simulink model "controller_v12_pagani_zonda_R"  (R2022b)
settings: Solver=ode4  StartTime=0.0  StopTime=10  FixedStep=0.00001  RelTol=1e-3
values from neighbouring files (symbols this model uses):
  m = 6    [coordinator_v2.m]
  N = 10    [coordinator_v2.m]
undefined symbols (not defined in the file or in its folder): PD_result, sd, X, Y, Z
libraries: sm_lib x235, nesl_utility x83
(part 5 of 5)

== system controller_v12_pagani_zonda_R/Subsystem/base ==
  ReferenceFrame : sm_lib/Frames and Transforms/Reference Frame
  Visual : sm_lib/Body Elements/Brick Solid  GraphicAmbientColor=[0.15 0.15 0.15 1.0]  BasedOnType=Density  BrickDimensions=[0.001, 0.001, 0.001]  BrickDimensionUnits=m  CenterOfMass=[0, 0, 0]  CenterOfMassUnits=m  GraphicDiffuseColor=[0.5, 0.5, 0.5]  Density=1000  DensityUnits=kg/m^3  DoExposeReferenceFrame=on  GraphicEmissiveColor=[0.0 0.0 0.0 1.0]  ExportEntireGeometry=off  SerializedFrames=<Frames/>  MarkerShape=Sphere  MarkerSize=10  GraphicType=FromGeometry  InertiaType=Custom  Mass=0  MassUnits=kg  MomentsOfInertia=[0, 0, 0]  MomentsOfInertiaUnits=kg*m^2  GraphicOpacity=1  ProductsOfInertia=[0, 0, 0]  ProductsOfInertiaUnits=kg*m^2  GraphicShininess=75  GraphicSpecularColor=[0.5 0.5 0.5 1.0]  GraphicVisPropType=SimpleVisualProperties
  VisualOriginTransform : sm_lib/Frames and Transforms/Rigid Transform  TranslationMethod=Cartesian  TranslationStandardOffset=0  TranslationLengthUnit=m  TranslationStandardAxis=+Z  TranslationCartesianOffset=[0, 0, 0]  TranslationROffset=0  TranslationROffsetUnits=m  TranslationZOffset=0  TranslationZOffsetUnits=m  TranslationThetaOffset=0  TranslationThetaOffsetUnits=deg  RotationMethod=RotationSequence  RotationAngleUnits=deg  RotationStandardAxis=+Z  RotationAngle=0.0  RotationArbitraryAxis=[0 0 1]  FollAlignAxisA=+X  BaseAlignAxisA=+Y  FollAlignAxisB=+Y  BaseAlignAxisB=+Z  RotationSequenceAxes=BaseAxes  RotationSequence=XYZ  RotationSequenceAngles=[0, 0, 0]  RotationSequenceAnglesUnits=rad  RotationMatrix=[1 0 0; 0 1 0; 0 0 1]  Quaternion=[1 0 0 0]
  floating_base_OriginTransform : sm_lib/Frames and Transforms/Rigid Transform  TranslationMethod=Cartesian  TranslationStandardOffset=0  TranslationLengthUnit=m  TranslationStandardAxis=+Z  TranslationCartesianOffset=[0, 0, 0]  TranslationROffset=0  TranslationROffsetUnits=m  TranslationZOffset=0  TranslationZOffsetUnits=m  TranslationThetaOffset=0  TranslationThetaOffsetUnits=deg  RotationMethod=RotationSequence  RotationAngleUnits=deg  RotationStandardAxis=+Z  RotationAngle=0.0  RotationArbitraryAxis=[0 0 1]  FollAlignAxisA=+X  BaseAlignAxisA=+Y  FollAlignAxisB=+Y  BaseAlignAxisB=+Z  RotationSequenceAxes=BaseAxes  RotationSequence=XYZ  RotationSequenceAngles=[0, 0, 0]  RotationSequenceAnglesUnits=rad  RotationMatrix=[1 0 0; 0 1 0; 0 0 1]  Quaternion=[1 0 0 0]
  F : PMIOPort  Side=Left
  F1 : PMIOPort  Port=2  Side=Right
  connections:
  VisualOriginTransform/LConn1 -- ReferenceFrame/RConn1 -- F/RConn1 -- floating_base_OriginTransform/LConn1
  Visual/RConn1 -- VisualOriginTransform/RConn1
  floating_base_OriginTransform/RConn1 -- F1/RConn1

== system controller_v12_pagani_zonda_R/Subsystem/imu_link ==
  Inertia : sm_lib/Body Elements/Inertia  InertiaType=Custom  Mass=0.001  MassUnits=kg  CenterOfMass=[0, 0, 0]  CenterOfMassUnits=m  MomentsOfInertia=[0.0001, 0.0001, 0.0001]  MomentsOfInertiaUnits=kg*m^2  ProductsOfInertia=[0, 0, 0]  ProductsOfInertiaUnits=kg*m^2  GraphicType=None  MarkerShape=Inertia  MarkerSize=20  GraphicVisPropType=SimpleVisualProperties  GraphicDiffuseColor=[0.5 0.5 0.5]  GraphicSpecularColor=[0.5 0.5 0.5 1.0]  GraphicAmbientColor=[0.15 0.15 0.15 1.0]  GraphicEmissiveColor=[0.0 0.0 0.0 1.0]  GraphicShininess=75  GraphicOpacity=1.0
  InertiaOriginTransform : sm_lib/Frames and Transforms/Rigid Transform  TranslationMethod=Cartesian  TranslationStandardOffset=0  TranslationLengthUnit=m  TranslationStandardAxis=+Z  TranslationCartesianOffset=[0, 0, 0]  TranslationROffset=0  TranslationROffsetUnits=m  TranslationZOffset=0  TranslationZOffsetUnits=m  TranslationThetaOffset=0  TranslationThetaOffsetUnits=deg  RotationMethod=RotationSequence  RotationAngleUnits=deg  RotationStandardAxis=+Z  RotationAngle=0.0  RotationArbitraryAxis=[0 0 1]  FollAlignAxisA=+X  BaseAlignAxisA=+Y  FollAlignAxisB=+Y  BaseAlignAxisB=+Z  RotationSequenceAxes=BaseAxes  RotationSequence=XYZ  RotationSequenceAngles=[0, 0, 0]  RotationSequenceAnglesUnits=rad  RotationMatrix=[1 0 0; 0 1 0; 0 0 1]  Quaternion=[1 0 0 0]
  ReferenceFrame : sm_lib/Frames and Transforms/Reference Frame
  Visual : sm_lib/Body Elements/Brick Solid  GraphicAmbientColor=[0.15 0.15 0.15 1.0]  BasedOnType=Density  BrickDimensions=[0.001, 0.001, 0.001]  BrickDimensionUnits=m  CenterOfMass=[0, 0, 0]  CenterOfMassUnits=m  GraphicDiffuseColor=[0.8, 0, 0]  Density=1000  DensityUnits=kg/m^3  DoExposeReferenceFrame=on  GraphicEmissiveColor=[0.0 0.0 0.0 1.0]  ExportEntireGeometry=off  SerializedFrames=<Frames/>  MarkerShape=Sphere  MarkerSize=10  GraphicType=FromGeometry  InertiaType=Custom  Mass=0  MassUnits=kg  MomentsOfInertia=[0, 0, 0]  MomentsOfInertiaUnits=kg*m^2  GraphicOpacity=1  ProductsOfInertia=[0, 0, 0]  ProductsOfInertiaUnits=kg*m^2  GraphicShininess=75  GraphicSpecularColor=[0.5 0.5 0.5 1.0]  GraphicVisPropType=SimpleVisualProperties
  VisualOriginTransform : sm_lib/Frames and Transforms/Rigid Transform  TranslationMethod=Cartesian  TranslationStandardOffset=0  TranslationLengthUnit=m  TranslationStandardAxis=+Z  TranslationCartesianOffset=[0, 0, 0]  TranslationROffset=0  TranslationROffsetUnits=m  TranslationZOffset=0  TranslationZOffsetUnits=m  TranslationThetaOffset=0  TranslationThetaOffsetUnits=deg  RotationMethod=RotationSequence  RotationAngleUnits=deg  RotationStandardAxis=+Z  RotationAngle=0.0  RotationArbitraryAxis=[0 0 1]  FollAlignAxisA=+X  BaseAlignAxisA=+Y  FollAlignAxisB=+Y  BaseAlignAxisB=+Z  RotationSequenceAxes=BaseAxes  RotationSequence=XYZ  RotationSequenceAngles=[0, 0, 0]  RotationSequenceAnglesUnits=rad  RotationMatrix=[1 0 0; 0 1 0; 0 0 1]  Quaternion=[1 0 0 0]
  F : PMIOPort  Side=Left
  connections:
  Inertia/RConn1 -- InertiaOriginTransform/RConn1
  ReferenceFrame/RConn1 -- InertiaOriginTransform/LConn1 -- VisualOriginTransform/LConn1 -- F/RConn1
  Visual/RConn1 -- VisualOriginTransform/RConn1

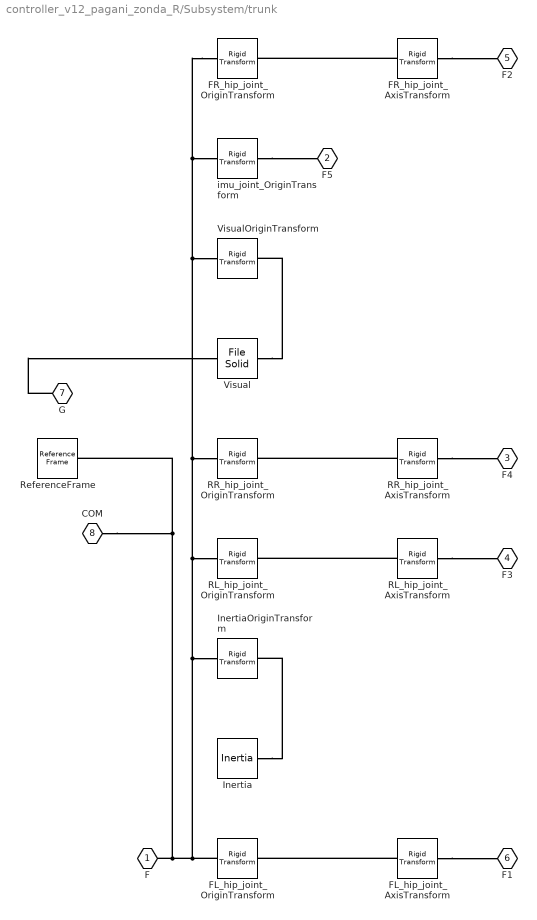
== system controller_v12_pagani_zonda_R/Subsystem/trunk ==
  FL_hip_joint_AxisTransform : sm_lib/Frames and Transforms/Rigid Transform  TranslationMethod=Cartesian  TranslationStandardOffset=0  TranslationLengthUnit=m  TranslationStandardAxis=+Z  TranslationCartesianOffset=[0, 0, 0]  TranslationROffset=0  TranslationROffsetUnits=m  TranslationZOffset=0  TranslationZOffsetUnits=m  TranslationThetaOffset=0  TranslationThetaOffsetUnits=deg  RotationMethod=ArbitraryAxis  RotationAngleUnits=rad  RotationStandardAxis=+Z  RotationAngle=1.570796326794897  RotationArbitraryAxis=[-0, 1, 0]  FollAlignAxisA=+X  BaseAlignAxisA=+Y  FollAlignAxisB=+Y  BaseAlignAxisB=+Z  RotationSequenceAxes=FollowerAxes  RotationSequence=XYX  RotationSequenceAngles=[0 0 0]  RotationSequenceAnglesUnits=deg  RotationMatrix=[1 0 0; 0 1 0; 0 0 1]  Quaternion=[1 0 0 0]
  FL_hip_joint_OriginTransform : sm_lib/Frames and Transforms/Rigid Transform  TranslationMethod=Cartesian  TranslationStandardOffset=0  TranslationLengthUnit=m  TranslationStandardAxis=+Z  TranslationCartesianOffset=[0.1805, 0.047, 0]  TranslationROffset=0  TranslationROffsetUnits=m  TranslationZOffset=0  TranslationZOffsetUnits=m  TranslationThetaOffset=0  TranslationThetaOffsetUnits=deg  RotationMethod=RotationSequence  RotationAngleUnits=deg  RotationStandardAxis=+Z  RotationAngle=0.0  RotationArbitraryAxis=[0 0 1]  FollAlignAxisA=+X  BaseAlignAxisA=+Y  FollAlignAxisB=+Y  BaseAlignAxisB=+Z  RotationSequenceAxes=BaseAxes  RotationSequence=XYZ  RotationSequenceAngles=[0, 0, 0]  RotationSequenceAnglesUnits=rad  RotationMatrix=[1 0 0; 0 1 0; 0 0 1]  Quaternion=[1 0 0 0]
  FR_hip_joint_AxisTransform : sm_lib/Frames and Transforms/Rigid Transform  TranslationMethod=Cartesian  TranslationStandardOffset=0  TranslationLengthUnit=m  TranslationStandardAxis=+Z  TranslationCartesianOffset=[0, 0, 0]  TranslationROffset=0  TranslationROffsetUnits=m  TranslationZOffset=0  TranslationZOffsetUnits=m  TranslationThetaOffset=0  TranslationThetaOffsetUnits=deg  RotationMethod=ArbitraryAxis  RotationAngleUnits=rad  RotationStandardAxis=+Z  RotationAngle=1.570796326794897  RotationArbitraryAxis=[-0, 1, 0]  FollAlignAxisA=+X  BaseAlignAxisA=+Y  FollAlignAxisB=+Y  BaseAlignAxisB=+Z  RotationSequenceAxes=FollowerAxes  RotationSequence=XYX  RotationSequenceAngles=[0 0 0]  RotationSequenceAnglesUnits=deg  RotationMatrix=[1 0 0; 0 1 0; 0 0 1]  Quaternion=[1 0 0 0]
  FR_hip_joint_OriginTransform : sm_lib/Frames and Transforms/Rigid Transform  TranslationMethod=Cartesian  TranslationStandardOffset=0  TranslationLengthUnit=m  TranslationStandardAxis=+Z  TranslationCartesianOffset=[0.1805, -0.047, 0]  TranslationROffset=0  TranslationROffsetUnits=m  TranslationZOffset=0  TranslationZOffsetUnits=m  TranslationThetaOffset=0  TranslationThetaOffsetUnits=deg  RotationMethod=RotationSequence  RotationAngleUnits=deg  RotationStandardAxis=+Z  RotationAngle=0.0  RotationArbitraryAxis=[0 0 1]  FollAlignAxisA=+X  BaseAlignAxisA=+Y  FollAlignAxisB=+Y  BaseAlignAxisB=+Z  RotationSequenceAxes=BaseAxes  RotationSequence=XYZ  RotationSequenceAngles=[0, 0, 0]  RotationSequenceAnglesUnits=rad  RotationMatrix=[1 0 0; 0 1 0; 0 0 1]  Quaternion=[1 0 0 0]
  Inertia : sm_lib/Body Elements/Inertia  InertiaType=Custom  Mass=6  MassUnits=kg  CenterOfMass=[0, 0, 0]  CenterOfMassUnits=m  MomentsOfInertia=[0.0158533, 0.0377999, 0.0456542]  MomentsOfInertiaUnits=kg*m^2  ProductsOfInertia=[-2.75e-05, -6.109999999999999e-05, -3.66e-05]  ProductsOfInertiaUnits=kg*m^2  GraphicType=None  MarkerShape=Inertia  MarkerSize=20  GraphicVisPropType=SimpleVisualProperties  GraphicDiffuseColor=[0.5 0.5 0.5]  GraphicSpecularColor=[0.5 0.5 0.5 1.0]  GraphicAmbientColor=[0.15 0.15 0.15 1.0]  GraphicEmissiveColor=[0.0 0.0 0.0 1.0]  GraphicShininess=75  GraphicOpacity=1.0
  InertiaOriginTransform : sm_lib/Frames and Transforms/Rigid Transform  TranslationMethod=Cartesian  TranslationStandardOffset=0  TranslationLengthUnit=m  TranslationStandardAxis=+Z  TranslationCartesianOffset=[0, 0.0041, -0.0005]  TranslationROffset=0  TranslationROffsetUnits=m  TranslationZOffset=0  TranslationZOffsetUnits=m  TranslationThetaOffset=0  TranslationThetaOffsetUnits=deg  RotationMethod=RotationSequence  RotationAngleUnits=deg  RotationStandardAxis=+Z  RotationAngle=0.0  RotationArbitraryAxis=[0 0 1]  FollAlignAxisA=+X  BaseAlignAxisA=+Y  FollAlignAxisB=+Y  BaseAlignAxisB=+Z  RotationSequenceAxes=BaseAxes  RotationSequence=XYZ  RotationSequenceAngles=[0, 0, 0]  RotationSequenceAnglesUnits=rad  RotationMatrix=[1 0 0; 0 1 0; 0 0 1]  Quaternion=[1 0 0 0]
  RL_hip_joint_AxisTransform : sm_lib/Frames and Transforms/Rigid Transform  TranslationMethod=Cartesian  TranslationStandardOffset=0  TranslationLengthUnit=m  TranslationStandardAxis=+Z  TranslationCartesianOffset=[0, 0, 0]  TranslationROffset=0  TranslationROffsetUnits=m  TranslationZOffset=0  TranslationZOffsetUnits=m  TranslationThetaOffset=0  TranslationThetaOffsetUnits=deg  RotationMethod=ArbitraryAxis  RotationAngleUnits=rad  RotationStandardAxis=+Z  RotationAngle=1.570796326794897  RotationArbitraryAxis=[-0, 1, 0]  FollAlignAxisA=+X  BaseAlignAxisA=+Y  FollAlignAxisB=+Y  BaseAlignAxisB=+Z  RotationSequenceAxes=FollowerAxes  RotationSequence=XYX  RotationSequenceAngles=[0 0 0]  RotationSequenceAnglesUnits=deg  RotationMatrix=[1 0 0; 0 1 0; 0 0 1]  Quaternion=[1 0 0 0]
  RL_hip_joint_OriginTransform : sm_lib/Frames and Transforms/Rigid Transform  TranslationMethod=Cartesian  TranslationStandardOffset=0  TranslationLengthUnit=m  TranslationStandardAxis=+Z  TranslationCartesianOffset=[-0.1805, 0.047, 0]  TranslationROffset=0  TranslationROffsetUnits=m  TranslationZOffset=0  TranslationZOffsetUnits=m  TranslationThetaOffset=0  TranslationThetaOffsetUnits=deg  RotationMethod=RotationSequence  RotationAngleUnits=deg  RotationStandardAxis=+Z  RotationAngle=0.0  RotationArbitraryAxis=[0 0 1]  FollAlignAxisA=+X  BaseAlignAxisA=+Y  FollAlignAxisB=+Y  BaseAlignAxisB=+Z  RotationSequenceAxes=BaseAxes  RotationSequence=XYZ  RotationSequenceAngles=[0, 0, 0]  RotationSequenceAnglesUnits=rad  RotationMatrix=[1 0 0; 0 1 0; 0 0 1]  Quaternion=[1 0 0 0]
  RR_hip_joint_AxisTransform : sm_lib/Frames and Transforms/Rigid Transform  TranslationMethod=Cartesian  TranslationStandardOffset=0  TranslationLengthUnit=m  TranslationStandardAxis=+Z  TranslationCartesianOffset=[0, 0, 0]  TranslationROffset=0  TranslationROffsetUnits=m  TranslationZOffset=0  TranslationZOffsetUnits=m  TranslationThetaOffset=0  TranslationThetaOffsetUnits=deg  RotationMethod=ArbitraryAxis  RotationAngleUnits=rad  RotationStandardAxis=+Z  RotationAngle=1.570796326794897  RotationArbitraryAxis=[-0, 1, 0]  FollAlignAxisA=+X  BaseAlignAxisA=+Y  FollAlignAxisB=+Y  BaseAlignAxisB=+Z  RotationSequenceAxes=FollowerAxes  RotationSequence=XYX  RotationSequenceAngles=[0 0 0]  RotationSequenceAnglesUnits=deg  RotationMatrix=[1 0 0; 0 1 0; 0 0 1]  Quaternion=[1 0 0 0]
  RR_hip_joint_OriginTransform : sm_lib/Frames and Transforms/Rigid Transform  TranslationMethod=Cartesian  TranslationStandardOffset=0  TranslationLengthUnit=m  TranslationStandardAxis=+Z  TranslationCartesianOffset=[-0.1805, -0.047, 0]  TranslationROffset=0  TranslationROffsetUnits=m  TranslationZOffset=0  TranslationZOffsetUnits=m  TranslationThetaOffset=0  TranslationThetaOffsetUnits=deg  RotationMethod=RotationSequence  RotationAngleUnits=deg  RotationStandardAxis=+Z  RotationAngle=0.0  RotationArbitraryAxis=[0 0 1]  FollAlignAxisA=+X  BaseAlignAxisA=+Y  FollAlignAxisB=+Y  BaseAlignAxisB=+Z  RotationSequenceAxes=BaseAxes  RotationSequence=XYZ  RotationSequenceAngles=[0, 0, 0]  RotationSequenceAnglesUnits=rad  RotationMatrix=[1 0 0; 0 1 0; 0 0 1]  Quaternion=[1 0 0 0]
  ReferenceFrame : sm_lib/Frames and Transforms/Reference Frame
  Visual : sm_lib/Body Elements/File Solid  ExtGeomFileName=a1_description\meshes\trunk.stl  UnitType=Custom  ExtGeomFileUnits=m  StepReaderType=HEX  ExportConvexHullGeometry=on  InertiaType=Custom  Mass=0  MassUnits=kg  CenterOfMass=[0, 0, 0]  CenterOfMassUnits=m  MomentsOfInertia=[0, 0, 0]  MomentsOfInertiaUnits=kg*m^2  ProductsOfInertia=[0, 0, 0]  ProductsOfInertiaUnits=kg*m^2  BasedOnType=DensityFromFile  Density=1000  DensityUnits=kg/m^3  DoExposeReferenceFrame=on  SerializedFrames=<Frames/>  GraphicType=FromGeometry  MarkerShape=Sphere  MarkerSize=10  GraphicVisPropType=SimpleVisualProperties  GraphicDiffuseColor=[1, 0.423529411765, 0.0392156862745]  GraphicSpecularColor=[0.5 0.5 0.5 1.0]  GraphicAmbientColor=[0.15 0.15 0.15 1.0]  GraphicEmissiveColor=[0.0 0.0 0.0 1.0]  GraphicShininess=75  GraphicOpacity=1
  VisualOriginTransform : sm_lib/Frames and Transforms/Rigid Transform  TranslationMethod=Cartesian  TranslationStandardOffset=0  TranslationLengthUnit=m  TranslationStandardAxis=+Z  TranslationCartesianOffset=[0, 0, 0]  TranslationROffset=0  TranslationROffsetUnits=m  TranslationZOffset=0  TranslationZOffsetUnits=m  TranslationThetaOffset=0  TranslationThetaOffsetUnits=deg  RotationMethod=RotationSequence  RotationAngleUnits=deg  RotationStandardAxis=+Z  RotationAngle=0.0  RotationArbitraryAxis=[0 0 1]  FollAlignAxisA=+X  BaseAlignAxisA=+Y  FollAlignAxisB=+Y  BaseAlignAxisB=+Z  RotationSequenceAxes=BaseAxes  RotationSequence=XYZ  RotationSequenceAngles=[0, 0, 0]  RotationSequenceAnglesUnits=rad  RotationMatrix=[1 0 0; 0 1 0; 0 0 1]  Quaternion=[1 0 0 0]
  imu_joint_OriginTransform : sm_lib/Frames and Transforms/Rigid Transform  TranslationMethod=Cartesian  TranslationStandardOffset=0  TranslationLengthUnit=m  TranslationStandardAxis=+Z  TranslationCartesianOffset=[0, 0, 0]  TranslationROffset=0  TranslationROffsetUnits=m  TranslationZOffset=0  TranslationZOffsetUnits=m  TranslationThetaOffset=0  TranslationThetaOffsetUnits=deg  RotationMethod=RotationSequence  RotationAngleUnits=deg  RotationStandardAxis=+Z  RotationAngle=0.0  RotationArbitraryAxis=[0 0 1]  FollAlignAxisA=+X  BaseAlignAxisA=+Y  FollAlignAxisB=+Y  BaseAlignAxisB=+Z  RotationSequenceAxes=BaseAxes  RotationSequence=XYZ  RotationSequenceAngles=[0, 0, 0]  RotationSequenceAnglesUnits=rad  RotationMatrix=[1 0 0; 0 1 0; 0 0 1]  Quaternion=[1 0 0 0]
  F : PMIOPort  Side=Left
  F5 : PMIOPort  Port=2  Side=Right
  F4 : PMIOPort  Port=3  Side=Right
  F3 : PMIOPort  Port=4  Side=Right
  F2 : PMIOPort  Port=5  Side=Right
  F1 : PMIOPort  Port=6  Side=Right
  G : PMIOPort  Port=7  Side=Right
  COM : PMIOPort  Port=8  Side=Right
  connections:
  FL_hip_joint_AxisTransform/RConn1 -- F1/RConn1
  FL_hip_joint_AxisTransform/LConn1 -- FL_hip_joint_OriginTransform/RConn1
  FR_hip_joint_AxisTransform/RConn1 -- F2/RConn1
  FR_hip_joint_AxisTransform/LConn1 -- FR_hip_joint_OriginTransform/RConn1
  Inertia/RConn1 -- InertiaOriginTransform/RConn1
  RL_hip_joint_AxisTransform/RConn1 -- F3/RConn1
  RL_hip_joint_AxisTransform/LConn1 -- RL_hip_joint_OriginTransform/RConn1
  RR_hip_joint_AxisTransform/RConn1 -- F4/RConn1
  RR_hip_joint_AxisTransform/LConn1 -- RR_hip_joint_OriginTransform/RConn1
  FR_hip_joint_OriginTransform/LConn1 -- FL_hip_joint_OriginTransform/LConn1 -- COM/RConn1 -- ReferenceFrame/RConn1 -- F/RConn1 -- InertiaOriginTransform/LConn1 -- RL_hip_joint_OriginTransform/LConn1 -- RR_hip_joint_OriginTransform/LConn1 -- VisualOriginTransform/LConn1 -- imu_joint_OriginTransform/LConn1
  Visual/RConn1 -- VisualOriginTransform/RConn1
  imu_joint_OriginTransform/RConn1 -- F5/RConn1
  G/RConn1 -- Visual/LConn1

== matlab function controller_v12_pagani_zonda_R/MATLAB Function ==
  data: q1 input; q2 input; q3 input; q4 input; q5 input; q6 input; q7 input; q8 input; q9 input; q10 input; q11 input; q12 input; w1 input; w2 input; w3 input; w4 input; w5 input; w6 input; w7 input; w8 input; w9 input; w10 input; w11 input; w12 input; ss input; rr input; rl input; fr input; fl input; t input; u1 output; u2 output; u3 output; u4 output; u5 output; u6 output; u7 output; u8 output; u9 output; u10 output; u11 output; u12 output; vrr input; vrl input; vfr input; vfl input; last_MPC_result input; last_PD_result input; update_MPC_result output; MPC_thred input; update_MPC_thred output; update_PD_result output; PD_thred input; update_PD_thred output; sd input; update_sd output
function [u1, u2, u3, u4, u5, u6, u7, u8, u9, u10, u11, u12, update_MPC_result, update_MPC_thred, update_PD_result, update_PD_thred, update_sd] = coordinator(q1, q2, q3, q4, q5, q6, q7, q8, q9, q10, q11, q12, w1, w2, w3, w4, w5, w6, w7, w8, w9, w10, w11, w12, ss, rr, rl, fr, fl, t, vrr, vrl, vfr, vfl, last_MPC_result, last_PD_result, MPC_thred, PD_thred, sd)
    stand_interval = [0; 2];
    q = [q1;q2;q3;q4;q5;q6;q7;q8;q9;q10;q11;q12]; % Joint variable
    cur_time = t - stand_interval(2); % relative time bw world time and standing end time
    N = 10;
    dt = 0.05;
    dt_pd = 0.25;
    v_d = 0.5;
    robot_height = 0.3;
    p_direction = [1; 0; 0]; % direction of movement, must have x^2 + y^2 + z^2 = 1
    update_MPC_thred = MPC_thred;
    update_PD_thred = PD_thred;
    update_sd = sd;

    if cur_time < 0 % running pd controller for standing
        [u1,u2,u3,u4,u5,u6,u7,u8,u9,u10,u11,u12] = PD_constrol_standing(t,q1,q2,q3,q4,q5,q6,q7,q8,q9,q10,q11,q12,w1,w2,w3,w4,w5,w6,w7,w8,w9,w10,w11,w12);
        update_MPC_result = zeros(12, 1);
        update_PD_result = zeros(24, 10);
    else % running mpc controller for nbody motion and PD controller for swing legs after standing period
        if cur_time >= MPC_thred % update foot force every dt after standing end time
            update_MPC_thred = MPC_thred + dt;
            r = [fl; fr; rl; rr]; % Current foot position
%             sd = [0.1902;-0.0072; 0.29; 0; 0; 0; 0; 0; 0; 0; 0; 0; 9.81];
%             sd(7:9) = v_d * p_direction;
%             sd(1:3) = sd(1:3) + (v_d * p_direction) * dt;
%             update_sd = sd;
            sd = updatesd(ss, sd, t, v_d, p_direction, N, dt, robot_height, r);
            update_sd = sd;

            [update_MPC_result, modelist] = MPC_cntr_wrapper(ss, cur_time, r, dt, N, sd);
            y = update_MPC_result;
            [u1mpc,u2mpc,u3mpc,u4mpc,u5mpc,u6mpc,u7mpc,u8mpc,u9mpc,u10mpc,u11mpc,u12mpc] = force2torque(q,y,ss);
        else
            y = last_MPC_result;
            update_MPC_result = last_MPC_result;
            [u1mpc,u2mpc,u3mpc,u4mpc,u5mpc,u6mpc,u7mpc,u8mpc,u9mpc,u10mpc,u11mpc,u12mpc] = force2torque(q,y,ss);
        end

        n = 10; % number of division in swinging period.
        if cur_time >= PD_thred % Call PD function to swing leg every 0.15s
            update_PD_thred = PD_thred + dt_pd;
            r = [fl; fr; rl; rr]; % Current foot position
            vr = [vfl; vfr; vrl; vrr]; % current foot velovity
            [Pfoot_d,Vfoot_d] = get_Traj(cur_time, r, vr, ss, dt_pd, v_d, p_direction, n); % Calculate the desired position of foot at next period according to foot pos and COM pos & velo
            update_PD_result = [Pfoot_d;Vfoot_d]; % Update desired pos & velo for PD control
        else
            Pfoot_d = last_PD_result(1:12,:);
            Vfoot_d = last_PD_result(13:24,:);
            update_PD_result = last_PD_result;
            r = [fl; fr; rl; rr]; % Current foot position
            vr = [vfl; vfr; vrl; vrr]; % current foot velovity
        end

        i = floor(mod(cur_time,dt_pd)/0.025) + 1;

        iteration = floor(mod(cur_time/dt,N));
        if iteration < N/2 % foot 1, 4 on ground

            Pfoot_d(4:6,i) = next_foot_location(2, v_d * p_direction, r, N/2 * dt, n, (N/2), cur_time, N/2 * dt / n, ss);
            Pfoot_d(7:9,i) = next_foot_location(3, v_d * p_direction, r, N/2 * dt, n, N/2, cur_time, N/2 * dt / n, ss);
        else % foot 2, 3 on ground
            Pfoot_d(1:3,i) = next_foot_location(1, v_d * p_direction, r, N/2 * dt, n, N/2, cur_time, N/2 * dt / n, ss);
            Pfoot_d(10:12,i) = next_foot_location(4, v_d * p_direction, r, N/2 * dt, n, N/2, cur_time, N/2 * dt / n, ss);
        end
%         disp(Pfoot_d(:, i), [3, 4]);
%         disp(Vfoot_d(:, i), [3, 4]);
        F_swing = pd_control_for_leg_swing(Vfoot_d(:,i),Pfoot_d(:,i),r,vr); % Calculate the virtual force used for swing legs
        
%         if iteration < N/2 % foot 1, 4 on ground
%             F_swing(1:3) = zeros(3,1); % Forces applied on leg 1 is zero
%             F_swing(10:12) = zeros(3,1);
%         else % foot 2, 3 on ground
%             F_swing(4:6) = zeros(3,1); % Forces applied on leg 1 is zero
%             F_swing(7:9) = zeros(3,1);
%         end




        [u1pd, u2pd, u3pd, u4pd, u5pd, u6pd, u7pd, u8pd, u9pd, u10pd, u11pd, u12pd] = force2torque(q,F_swing,ss);
        
        
        u1 = u1mpc + u1pd;
        u2 = u2mpc + u2pd;
        u3 = u3mpc + u3pd;
        u4 = u4mpc + u4pd;
        u5 = u5mpc + u5pd;
        u6 = u6mpc + u6pd;
        u7 = u7mpc + u7pd;
        u8 = u8mpc + u8pd;
        u9 = u9mpc + u9pd;
        u10 = u10mpc + u10pd;
        u11 = u11mpc + u11pd;
        u12 = u12mpc + u12pd;
    end
end

%% desired system state update
function update = updatesd(ss, sd, t, v_d, p_direction, N, dt, robot_height, r)
        % change p_direction and baseline
        iteration = floor(mod(t/dt,N));
        if iteration < N/2
            front = r(1:3);
            rear = r(9:12);
            fheight = r(3);
            rheight = r(12);
        else
            front = r(4:6);
            rear = r(6:9);
            fheight = r(6);
            rheight = r(9);
        end
        angle = 0;
        if fheight - rheight > 0.1
            slope = (front(3) - rear(3)) / (front(1) - rear(1));
            angle = atan(slope) / 2;
%             sd(1) = (front(1) + rear(1)) / 2 - robot_height * sin(angle);
            sd(1) = (front(1) + rear(1)) / 2;
            sd(3) = robot_height * cos(angle) + (fheight + rheight) / 2;
            sd(5) = -angle;
%             disp(iteration < N/2);
%             disp(transpose(p_direction));
%             disp(transpose(sd));
%             disp(transpose(ss));
        end

        p_direction(1) = cos(angle);
        p_direction(2) = 0;
        p_direction(3) = sin(angle);
        % change sd base on direction
        if t > 1.06 
            sd(5) = -0.1;
        end
        sd(7:9) = [v_d; 0; v_d * tan(angle)];
        sd(1:3) = sd(1:3) + [v_d; 0; v_d * tan(angle)] * dt;
        update = sd;


end
%% PD controller for Standing
function [u1,u2,u3,u4,u5,u6,u7,u8,u9,u10,u11,u12] = PD_constrol_standing(t,q1,q2,q3,q4,q5,q6,q7,q8,q9,q10,q11,q12,w1,w2,w3,w4,w5,w6,w7,w8,w9,w10,w11,w12)
    kp1 = 100;
    kv1 = 40;
    kp2 = 120;
    kv2 = 50;

    q1d = 0; 
    q4d = 0;
    q7d = 0;
    q10d = 0;
    q2d = 0.78;
    q5d = 0.78;
    q8d = 0.78;
    q11d = 0.78;
    q3d = -1.57;
    q6d = -1.57;
    q9d = -1.57;
    q12d = -1.57;

     w1d = 0;
    w2d = 0;
    w3d = 0;
    w4d = 0;
    w5d = 0;
    w6d = 0;
    w7d = 0;
    w8d = 0;
    w9d = 0;
    w10d = 0;
    w11d = 0;
    w12d = 0;

    if t < 0.4
        u1 = 0;
        u2 = 0;
        u3 = 0;
        u4 = 0;
        u5 = 0;
        u6 = 0;
        u7 = 0;
        u8 = 0;
        u9 = 0;
        u10 = 0;
        u11 = 0;
        u12 = 0;
    
    else 
        u1 = kp2*(q1d-q1)+kv2*(w1d-w1);
        u2 = kp2*(q2d-q2)+kv2*(w2d-w2);
        u3 = kp2*(q3d-q3)+kv2*(w3d-w3);
        u4 = kp2*(q4d-q4)+kv2*(w4d-w4);
        u5 = kp2*(q5d-q5)+kv2*(w5d-w5);
        u6 = kp2*(q6d-q6)+kv2*(w6d-w6);
        u7 = kp1*(q7d-q7)+kv1*(w7d-w7);
        u8 = kp1*(q8d-q8)+kv1*(w8d-w8);
        u9 = kp1*(q9d-q9)+kv1*(w9d-w9);
        u10 = kp1*(q10d-q10)+kv1*(w10d-w10);
        u11 = kp1*(q11d-q11)+kv1*(w11d-w11);
        u12 = kp1*(q12d-q12)+kv1*(w12d-w12);
    end
end

%% MPC controller
% Input:
% System state: s, (12, 1)
% time: t
% mode: mode, indicating which foot on ground
% foot positions: r = [r_front_left; r_front_right; r_rear_left;
% r_rear_right]
% Inertial of body: Ib
% body mass: m
% time step: dt
% MPC horizon length: N
% Desired system state: sd
% Output:
% Foot force: y = [F_front_left; F_front_right; F_rear_left;
% F_rear_right]: 
% q: [x; y; z; roll; pitch; yaw; dx; dy; dz; w]
% sd: [xd; yd; zd; roll_d; pitch_d; yaw_d; dx_d; dy_d; dz_d; w_d]
% r: foot positions in world frame
%% Controller functions
% q: [x; y; z; roll; pitch; yaw; dx; dy; dz; w]
% sd: [xd; yd; zd; roll_d; pitch_d; yaw_d; dx_d; dy_d; dz_d; w_d]
% r: foot positions in world frame
function [y, mode_list] = MPC_cntr_wrapper(q, t, r, dt, N, sd)
    Ib = [0.0168, 0, 0;
        0, 0.0565, 0;
        0, 0, 0.064];
    m = 12;
    mode_list = zeros(N, 1);
    iteration = floor(mod(t/dt,N));
%     disp(t);
%     disp(iteration);
    
    for i = 0:N-1
        iter = mod((i + iteration), N);
        if iter < N / 2
            mode_list(i + 1) = 1;
        else
            mode_list(i + 1) = 2;
        end
    end
    y = -MPC_controller(q, t, mode_list, r, Ib, m, dt, N, sd);
end

function y = MPC_controller(q, t, mode_list, r, Ib, m, dt, N, sd)
    p = q(1:3);
    eul = q(4:6);
    dp = q(7:9);
    wb = q(10:12);
    
    r1 = r(1:3) - p;
    r2 = r(4:6) - p;
    r3 = r(7:9) - p;
    r4 = r(10:12) - p;
    xd = sd;
    Q_mpc = diag([40,50,6000,40000,60000,40,4,4,4,1,1,1]);
    R_mpc = 0.000001 * eye(12);

    state_num = 13;
    controller_num = 12;
    
    q0 = q;
    
    [Act, Bct]=linearize(q, [r1; r2; r3; r4], Ib, m, sd);
    
    Q_mpc = blkdiag(Q_mpc,0);
    xd = sd;
    
    QCell = repmat({Q_mpc}, 1, N);
    RCell = repmat({R_mpc}, 1, N);
    H = blkdiag(QCell{:}, RCell{:});
    f_blk = -Q_mpc*xd;
    f = [repmat(f_blk, N, 1);zeros(N*controller_num,1)];
    
    [Aeq, Beq] = get_equality_constraint([q0; 9.81], Act, Bct, dt, N);

    Aineq_right_size = zeros(N * 24, N * 12);
    Bineq = zeros(24 * N, 1);
    for i = 1:N
        mode = mode_list(i);
        if mode == 0
            [Ain, Bin] = MPC_all_foot();
            Ain_sz = size(Ain);
            start_row = 24 * (i-1) + 1;
            start_col = 12 * (i-1) + 1;
            Aineq_right_size(start_row : (Ain_sz(1) + start_row - 1), start_col : (Ain_sz(2) + start_col - 1)) = Ain;
            Bineq((24 * (i-1) + 1) : 24 * i) = Bin;
        elseif mode == 1
            [Ain, Bin] = MPC_fl_rr_foot();
            Ain_sz = size(Ain);
            start_row = 24 * (i-1) + 1;
            start_col = 12 * (i-1) + 1;
            Aineq_right_size(start_row : (Ain_sz(1) + start_row - 1), start_col : (Ain_sz(2) + start_col - 1)) = Ain;
            Bineq((24 * (i-1) + 1) : 24 * i) = Bin;
        elseif mode == 2
            [Ain, Bin] = MPC_fr_rl_foot();
            Ain_sz = size(Ain);
            start_row = 24 * (i-1) + 1;
            start_col = 12 * (i-1) + 1;
            Aineq_right_size(start_row : (Ain_sz(1) + start_row - 1), start_col : (Ain_sz(2) + start_col - 1)) = Ain;
            Bineq((24 * (i-1) + 1) : 24 * i) = Bin;
        elseif mode == 3
            [Ain, Bin] = MPC_f_foot();
            Ain_sz = size(Ain);
            start_row = 24 * (i-1) + 1;
            start_col = 12 * (i-1) + 1;
            Aineq_right_size(start_row : (Ain_sz(1) + start_row - 1), start_col : (Ain_sz(2) + start_col - 1)) = Ain;
            Bineq((24 * (i-1) + 1) : 24 * i) = Bin;
        elseif mode == 4
            [Ain, Bin] = MPC_r_foot();
            Ain_sz = size(Ain);
            start_row = 24 * (i-1) + 1;
            start_col = 12 * (i-1) + 1;
            Aineq_right_size(start_row : (Ain_sz(1) + start_row - 1), start_col : (Ain_sz(2) + start_col - 1)) = Ain;
            Bineq((24 * (i-1) + 1) : 24 * i) = Bin;
        end
    end

%     Aineq = [];
%     Bineq = [];
% 
%     for i=1:N
%         mode = mode_list(i);
%         if mode == 0
%             [Ain, Bin] = MPC_all_foot();
%             Aineq = blkdiag(Aineq, Ain);
%             Bineq = [Bineq; Bin];
%         elseif mode == 1
%             [Ain, Bin] = MPC_fl_rr_foot();
%             Aineq = blkdiag(Aineq, Ain);
%             Bineq = [Bineq; Bin];
%         elseif mode == 2
%             [Ain, Bin] = MPC_fr_rl_foot();
%             Aineq = blkdiag(Aineq, Ain);
%             Bineq = [Bineq; Bin];
%         elseif mode == 3
%             [Ain, Bin] = MPC_f_foot();
%             Aineq = blkdiag(Aineq, Ain);
%             Bineq = [Bineq; Bin];
%         elseif mode == 4
%             [Ain, Bin] = MPC_r_foot();
%             Aineq = blkdiag(Aineq, Ain);
%             Bineq = [Bineq; Bin];
%         end
%     end

    A_sz = size(Aineq_right_size);
    Aineq = [zeros(A_sz(1), state_num * N), Aineq_right_size];
    options = optimoptions('quadprog','Display','off', 'Algorithm','active-set');
    x0 = zeros(25 * N, 1);
    x0(1:12) = q0;
    x0(13) = 9.81;
    X_star = quadprog(H,f,Aineq,Bineq,Aeq,Beq,[],[],x0,options);

    y = X_star(N*state_num+1:N*state_num+controller_num);
end

% mode = 0, Four foot on ground
function [Ain, Bin] = MPC_all_foot()
    [A, B]=singleIneq();
    A_sz = size(A);
    Ain = A;
    Bin = B;
end

% mode = 1, front left and rear right on ground
function [Ain, Bin] = MPC_fl_rr_foot()
    [A, B]=singleIneq(); % F = [F1; F2; F3; F4], AF < B
    B(1 * 6 + 1) = 0;
    B(1 * 6 + 2) = 0;
    B(2 * 6 + 1) = 0;
    B(2 * 6 + 2) = 0;

    Ain = A;
    Bin = B;
end

% mode = 2, front right and rear left on ground
function [Ain, Bin] = MPC_fr_rl_foot()
    [A, B]=singleIneq();
    B(0 * 6 + 1) = 0;
    B(0 * 6 + 2) = 0;
    B(3 * 6 + 1) = 0;
    B(3 * 6 + 2) = 0;
    
    Ain = A;
    Bin = B;
end

% mode = 3, both front on ground
function [Ain, Bin] = MPC_f_foot()
    [A, B]=singleIneq();
    B(0 * 6 + 1) = 0;
    B(0 * 6 + 2) = 0;
    B(1 * 6 + 1) = 0;
    B(1 * 6 + 2) = 0;
    
    Ain = A;
    Bin = B;
end

% mode = 4, both rear on ground
function [Ain, Bin] = MPC_r_foot()
    [A, B]=singleIneq();
    B(2 * 6 + 1) = 0;
    B(2 * 6 + 2) = 0;
    B(3 * 6 + 1) = 0;
    B(3 * 6 + 2) = 0;
    
    Ain = A;
    Bin = B;
end

%% utility functions
% Transformation matrix to transform euler angle velocity to angular
% velocity
function T=Trans_euler2angular(Theta)
    theta = Theta(2);
    Phi = Theta(3);
    T = [cos(Phi) * cos(theta), -sin(Phi), 0;
        sin(Phi) * cos(theta), cos(Phi), 0;
        -sin(theta), 0, 1];
end

% Skew matrix from vector
function S = vector2skewmat(a)
    S = [0 -a(3) a(2);
     a(3) 0 -a(1);
     -a(2) a(1) 0];
end

% Matrix A, B in linearization
% input:
% System state: s
% Foot positions: r = [r_front_left; r_front_right; r_rear_left;
% r_rear_right]
% Inertial in world frame: Iw
% body mass: m
function [Act, Bct]=linearize(s, r, Ib, m, sd)
    p = s(1:3);
    eul = s(4:6);
    dp = s(7:9);
    wb = s(10:12);
    r1 = r(1:3);
    r2 = r(4:6);
    r3 = r(7:9);
    r4 = r(10:12);
    
    R = eul2rotm([eul(3), eul(2), eul(1)]);
    yaw = eul(3);
    Rz_yaw = [cos(yaw) sin(yaw) 0;
             -sin(yaw) cos(yaw) 0;
             0 0 1];
    Act = [zeros(3) zeros(3) eye(3) zeros(3) zeros(3,1);
             zeros(3) zeros(3) zeros(3) Rz_yaw zeros(3,1);
             zeros(3) zeros(3) zeros(3) zeros(3) [0;0;-1];
             zeros(4,13)];
    Iw = R'*Ib*R;
    D = [m*eye(3) zeros(3);
         zeros(3) Iw];
    A = [eye(3), eye(3), eye(3), eye(3);
        vector2skewmat(r1),vector2skewmat(r2),vector2skewmat(r3),vector2skewmat(r4)];
    Bct = [zeros(6,12);
             D\A;
             zeros(1,12)];

end

function [Aeq, Beq]=get_equality_constraint(s, A, B, dt, N)
    A_bar = A * dt + eye(size(A));
    B_bar = B * dt;

    ss = zeros(13, 1);
%     ss(1:12) = s;
%     ss(13) = 9.81;
    
    ss = s;

    Aside = eye(size(A) * N);
    sz = size(A);
    for i=2:N
        row_start = (i-1) * sz(1) + 1;
        row_end = i * sz(1);
        col_start = (i-2) * sz(2) + 1;
        col_end = (i-1) * sz(2);
        Aside(row_start:row_end, col_start:col_end) = -A_bar;
    end

    BCell = repmat({-B_bar}, 1, N);
    Bside = blkdiag(BCell{:});
    Aeq = [Aside, Bside];
    Beq = zeros(N * 13, 1);
    Beq(1:13) = A_bar * ss;
end

% F = [F1; F2; F3; F4] inequality constraint
function [A, B]=singleIneq()
    mu = 0.5;
    a = [0, 0, 1;
        0, 0, -1;
        1, 0, -mu;
        -1, 0, -mu;
        0, 1, -mu;
        0, -1, -mu];
    b = [500; -10; 0; 0; 0; 0];
    A = blkdiag(a, a, a, a);
    B = [b; b; b; b];
end

%% Foot Trajectory
function [Position_d, Velocity_d] = FootTraj_forward(Pfoot_c, q, dt, v_d, p_direction, leg, n)
% This function will given a series of desired pos and velo for one foot in the following time period, each foot needs a trajectory and velovity should call this function seperately
% Input: Pfoot_c: the rcurrent position of this foot

% Sign for translatio between COM and hip: FL: ++; FR: +-; RL: -+; RR: --.
if leg == 1 || leg == 2
    sidesign1 = 1;
else 
    sidesign1 = -1;
end

if leg == 1 || leg == 3
    sidesign2 = 1;
else
    sidesign2 = -1;
end
p_COM = q(1:3); % Current position of COM
v_COM = q(7:9); % Velocity of COM
R = eul2rotm([q(6), q(5), q(4)]); % Rotation matrix of trunk
d = [sidesign1*0.1335; sidesign2*0.097; 0]; % Translation from COM to hip
Phip_p = p_COM + v_COM*dt + R*d; % predicted pos of hip 

g = 9.81; % gravity
K_step = sqrt(p_COM(3)/g); % The coefficient of feedback

v_forward = v_d*p_direction; % desired velocity of walking forward
Pfoot_pre = [Phip_p(1:2); Pfoot_c(3)] + (dt/2) * v_COM + K_step * (v_COM - v_forward); % predict foot position at next dt instant
d = Pfoot_pre-Pfoot_c; % vector from current foot position to predicted foot position
t = linspace(0,dt,11); % cut one time period in 10 segments

wz = 2*pi/dt; % angular frequency for trig function in z direction
Az = wz*0.05/2; % amplitude
vz = Az*sin(wz*t); % function of vlocity in z direction
z = -Az/wz*cos(wz*t) + Az/wz; % function of trajection in z direction

wxy = pi/dt; % angular frequency for trig function in x&y direction
Ax = d(1)*wxy/2;
vx = Ax*sin(wxy*t);
x = -Ax/wxy*cos(wxy*t) + Ax/wxy;

Ay = d(2)*wxy/2;
vy = Ay*sin(wxy*t);
y = -Ay/wxy*cos(wxy*t) + Ay/wxy;



Position_d = [x(2:end); y(2:end); z(2:end)] + Pfoot_c; % output1: the desired position of this foot in the world frame, 3x10
Velocity_d = [vx(2:end); vy(2:end); vz(2:end)]; % output2: the desired velo of this foot in the world frame, 3x10
end


function y = pd_control_for_leg_swing(Vfoot_d,Pfoot_d,r,vr)
% PD control for calculating leg swing force 
% Inputs: Vfoot_d - desired velocity of all feet 12x1; Pfoot_d - desired
% position of all feet, 12x1; r - current pos of all feet, 12x1; vr -
% current velo of all feet, 12x1;
% NOTE: The sequence is [FL; FR; RL; RR]

Kp_f = 300;
Kd_f = 50; % Kp & Kd for front leg
Kp_r = 200;
Kd_r = 30; % Kp & Kd for rear leg
y_f = Kp_f * (Pfoot_d(1:6) - r(1:6)) + Kd_f * (Vfoot_d(1:6) - vr(1:6)); % Swing forces applied on two front legs
y_r = Kp_r * (Pfoot_d(7:end) - r(7:end)) + Kd_r * (Vfoot_d(7:end) - vr(7:end)); % Swing forces applied on two rear legs
y = [y_f;y_r]; % Combine all forces applied on all legs together, 12x1
end

function [u1,u2,u3,u4,u5,u6,u7,u8,u9,u10,u11,u12] = force2torque(q,y,ss)
%Convert Force to joint torque,

% inputs are q(joint variable)
% Input Jacobian (left and right)
% Output u1 to u12, based on 细狗diagram plz refer to 细狗diagram


R=eul2rotm([ss(6),ss(5),ss(4)]);
Rt=transpose(R);
F1 = [y(1);y(2);y(3)];
F2 = [y(4);y(5);y(6)];
F3 = [y(7);y(8);y(9)];
F4 = [y(10);y(11);y(12)];


J_front_left = computeLegJacobianAndPosition([q(1); q(2); q(3)], 1);
J_front_right = computeLegJacobianAndPosition([q(4); q(5); q(6)], 2);
J_rear_left = computeLegJacobianAndPosition([q(7); q(8); q(9)], 3);
J_rear_right = computeLegJacobianAndPosition([q(10); q(11); q(12)], 4);
tauFL = transpose(J_front_left)*Rt*F1;
tauFR = transpose(J_front_right)*Rt*F2;
tauRL = transpose(J_rear_left)*Rt*F3;
tauRR = transpose(J_rear_right)*Rt*F4;

% u1 = tauFL(1);
% u2 = tauFL(2);
% u3 = tauFL(3);
% u4 = tauFR(1);
% u5 = tauFR(2);
% u6 = tauFR(3);
% u7 = tauLR(1);
% u8 = tauLR(2);
% u9 = tauLR(3);
% u10 = tauRR(1);
% u11 = tauRR(2);
% u12 = tauRR(3);
u1 = tauFL(1);
u2 = tauFL(2);
u3 = tauFL(3);
u4 = tauFR(1);
u5 = tauFR(2);
u6 = tauFR(3);
u7 = tauRL(1);
u8 = tauRL(2);
u9 = tauRL(3);
u10 = tauRR(1);
u11 = tauRR(2);
u12 = tauRR(3);
end

function [Pfoot_d,Vfoot_d] = get_Traj(cur_time, Pfoot_c, Vfoot_c, ss, dt_pd, v_d, p_direction, n)
% This function will find out which leg is swing leg and give the desired
% trajectory and velocity to that leg seperately. 
% Input: y - forces from MPC controller; Pfoot_c - current foot pos;
% Vfoot_c - current foot velocity; ss - system state (trunk); dt_pd - time
% of stance; v_d - desired speed; p_direction - moving direction; t - time 
% of staring PD;


p_fl = Pfoot_c(1:3);
p_fr = Pfoot_c(4:6);
p_rl = Pfoot_c(7:9);
p_rr = Pfoot_c(10:12);

v_fl = Vfoot_c(1:3);
v_fr = Vfoot_c(4:6);
v_rl = Vfoot_c(7:9);
v_rr = Vfoot_c(10:12);


if mod(cur_time,0.3) < 0.001 % mode 1, FL&RR stance; FR&RL swing
    Position_d_FL = repmat(p_fl,1,10); Velocity_d_FL = repmat(v_fl,1,10); % leg 1 (FL)
    [Position_d_FR, Velocity_d_FR] = FootTraj_forward(p_fr, ss, dt_pd, v_d, p_direction, 2, n); % leg 2 (FR)
    [Position_d_RL, Velocity_d_RL] = FootTraj_forward(p_rl, ss, dt_pd, v_d, p_direction, 3, n); % leg 3 (RL)
    Position_d_RR = repmat(p_rr,1,10); Velocity_d_RR = repmat(v_rr,1,10); % leg 4 (RR)
else % mode 2
    [Position_d_FL, Velocity_d_FL] = FootTraj_forward(p_fl, ss, dt_pd, v_d, p_direction, 1, n);
    Position_d_FR = repmat(p_fr,1,10); Velocity_d_FR = repmat(v_fr,1,10);
    Position_d_RL = repmat(p_rl,1,10); Velocity_d_RL = repmat(v_rl,1,10);
    [Position_d_RR, Velocity_d_RR] = FootTraj_forward(p_rr, ss, dt_pd, v_d, p_direction, 4, n); 
end


% if sqrt(sum(F_fl.^2)) < 0.01
%     leg = 1; % Front Left leg
%     [Position_d_FL, Velocity_d_FL] = FootTraj_forward(p_fl, ss, dt_pd, v_d, p_direction, leg, n); % If this leg is a swing leg, call function to calculate its desired pos and velo
% else
%     Position_d_FL = repmat(p_fl,1,10);
%     Velocity_d_FL = repmat(v_fl,1,10); % If this leg is not a swing leg, keeps its pos and velo as input
% end
% 
% if sqrt(sum(F_fr.^2)) < 0.01
%     leg = 2; % Front Right leg
%     [Position_d_FR, Velocity_d_FR] = FootTraj_forward(p_fr, ss, dt_pd, v_d, p_direction, leg, n);
% else
%     Position_d_FR = repmat(p_fr,1,10);
%     Velocity_d_FR = repmat(v_fr,1,10);
% end
% 
% if sqrt(sum(F_rl.^2)) < 0.01
%     leg = 3;
%     [Position_d_RL, Velocity_d_RL] = FootTraj_forward(p_rl, ss, dt_pd, v_d, p_direction, leg, n);
% else
%     Position_d_RL = repmat(p_rl,1,10);
%     Velocity_d_RL = repmat(v_rl,1,10);
% end
% 
% if sqrt(sum(F_rr.^2)) < 0.01
%     leg = 4;
%     [Position_d_RR, Velocity_d_RR] = FootTraj_forward(p_rr, ss, dt_pd, v_d, p_direction, leg, n); 
% else
%     Position_d_RR = repmat(p_rr,1,10);
%     Velocity_d_RR = repmat(v_rr,1,10);
% end
% disp(cur_time)
Pfoot_d = [Position_d_FL;Position_d_FR;Position_d_RL;Position_d_RR]; % output1: the desired pos for all feet, 12x10
% disp(Pfoot_d)
Vfoot_d = [Velocity_d_FL;Velocity_d_FR;Velocity_d_RL;Velocity_d_RR]; % output2: the desired velo for all feet, 12x10
end



function [F_FL,F_FR,FF_LR,F4_RR] = torque2force(q,u,ss)
%Convert Force to joint torque,

% inputs are q(joint variable)
% Input Jacobian (left and right)
% Output u1 to u12, based on 细狗diagram plz refer to 细狗diagram
tauFL = zeros(3,1);
tauFR = zeros(3,1);
tauLR = zeros(3,1);
tauRR = zeros(3,1);

tauFL(1) = u(1);
tauFL(2) = u(2);
tauFL(3) = u(3);
tauFR(1) = u(4);
tauFR(2) = u(5);
tauFR(3) = u(6);
tauLR(1) = u(7);
tauLR(2) = u(8);
tauLR(3) = u(9);
tauRR(1) = u(10);
tauRR(2) = u(11);
tauRR(3) = u(12);
R=eul2rotm([ss(6),ss(5),ss(4)]);

F_FL = R* inv(transpose(computeLegJacobianAndPosition([q(1); q(2); q(3)], 1))) *tauFL;
F_FR = R* inv(transpose(computeLegJacobianAndPosition([q(4); q(5); q(6)], 2))) *tauFR;
FF_LR = R* inv(transpose(computeLegJacobianAndPosition([q(7); q(8); q(9)], 3))) *tauLR;
F4_RR = R* inv(transpose(computeLegJacobianAndPosition([q(10); q(11); q(12)], 4))) *tauRR;

end

function J = computeLegJacobianAndPosition(q, leg)
    l1 = 0.045;
    l2 = 0.2;
    l3 = 0.2;
    
    if leg == 1 || leg == 3
        sideSign = 1;
    else
        sideSign = -1;
    end
    s1 = sin(q(1));
    s2 = sin(q(2));
    s3 = sin(q(3));
    c1 = cos(q(1));
    c2 = cos(q(2));
    c3 = cos(q(3));

    c23 = c2 * c3 - s2 * s3;
    s23 = s2 * c3 + c2 * s3;

    J = zeros(3, 3);
    J(1, 1) = 0;
    J(2, 1) = -sideSign * l1 * s1 + l2 * c2 * c1 + l3 * c23 * c1;
    J(3, 1) = sideSign * l1 * c1 + l2 * c2 * s1 + l3 * c23 * s1;
    J(1, 2) = -l3 * c23 - l2 * c2;
    J(2, 2) = -l2 * s2 * s1 - l3 * s23 * s1;
    J(3, 2) = l2 * s2 * c1 + l3 * s23 * c1;
    J(1, 3) = -l3 * c23;
    J(2, 3) = -l3 * s23 * s1;
    J(3, 3) = l3 * s23 * c1;
end

% timestep: time length for each stance stick of leg_index, like dt in mpc
% swing_ticks: number of updates for swing force in each swing
% phase_length: swinging time
% stance_ticks: number of updates for stance force when standing
function location = next_foot_location(leg_index, v_com, r, phase_length, swing_ticks, stance_ticks, ticks, time_step, ss)
  
    robot_height = -0.52;
    yaw_rate = 0;
    stair_dx = 0.2;
    stair_dz = 0.2;
    stair_start = 0.9;
    skip_range = stair_dx * 0.5;
    swing_prop = subphase_ticks(ticks, phase_length, time_step) / (swing_ticks);
    foot = r((3*(leg_index - 1) + 1):3*(leg_index));
    swing_height_ = swing_height(swing_prop);
    touchdown_location = raibert_touchdown_location(foot, v_com, stance_ticks, phase_length, time_step, yaw_rate, ss); % on x-y plane
    touchdown_location(3) = foot(3);

    dist2stairstep = stair_start - touchdown_location(1);
    stair_num = 0;
    while dist2stairstep < 0
        dist2stairstep = dist2stairstep + stair_dx;
        stair_num = stair_num + 1;
    end
    if dist2stairstep < skip_range
        touchdown_location(1) = touchdown_location(1) + skip_range;
    end

%     if touchdown_location(1) > stair_start - skip_range && foot(1) > stair_start - stair_dx
    if touchdown_location(1) > stair_start - stair_dx * 0.75
        swing_height_ = swing_height_ + stair_num * stair_dz + stair_dz * 1.2;
        disp(swing_height_);
    end

    time_left = time_step * swing_ticks * (1.0 - swing_prop);
    velocity = (touchdown_location - foot) / (time_left) .* [1; 1; 0];

    delta_foot_location = velocity * time_step;

    z_vector = [0; 0; swing_height_];

    location = foot .* [1; 1; 0] + z_vector + delta_foot_location;
end

function touchdown_location = raibert_touchdown_location(foot, v_d, stance_ticks, phase_length, time_step, yaw_rate, ss)
    v_com = ss(7:9);
    foot(3) = 0;
    delta_pos_2d = v_d * phase_length * time_step;
    delta_pos = [delta_pos_2d(1); delta_pos_2d(2); 0];
    theta = stance_ticks * time_step * yaw_rate;
    rotation = rotz(theta);
    Kstep = 0.02;
    delta_v = v_com - v_d;
    delta_v(3) = 0;
    touchdown_location = rotation * foot + delta_pos + Kstep * delta_v;
%     touchdown_location = rotation * foot + delta_pos;
end

function rz = rotz(gamma)
    rz = [cos(gamma), -sin(gamma), 0;
         sin(gamma), cos(gamma),  0;
         0,          0,           1];
end

% return which segment of swinging movement
function tick = subphase_ticks(ticks, phase_length, time_step)
    phase_time = mod(ticks, phase_length);
    tick =  floor(phase_time / time_step);
end

% expected moving height for current state
function swing_height_ = swing_height(swing_phase)
    z_leg_lift = 0.18;
    swing_height_ = z_leg_lift*sqrt(1 - (swing_phase - 0.5)^2 / 0.25);
end

function yes = isInStair(location, stair_dx, stair_dz, stair_start)
    x = location(1);
    y = location(2);
    z = location(3);
%     while stair_start < x
%         stair_start = stair_start + stair_dx;
%     end
%     if stair_start - x < stair_dx / 2
%         yes = 1;
%     else
%         yes = 0;
%     end

    stair_num = floor((x - stair_start) / stair_dx) + 1;
    if stair_num > 0 && stair_num * stair_dz > z
        yes = 1;
    else
        yes = 0;
    end
end
